simulink model "vr_octavia_graphs"  (Simulink 7.5)
settings: Solver=ode45  StartTime=0.0  StopTime=111.56  RelTol=1e-3
PostLoadFcn:
  | load octavia_testlap
undefined symbols (not defined in the file or in its folder): octavia_graphs
libraries: vrlib x26, simulink x1
Description:
  | Vehicle Dynamics Visualization with Graphs
  | 
  | This example extends the vr_octavia example and shows how combine virtual
  | reality canvas in one figure with other graphical user interface objects.
  | In this case, three graphs are displayed under the virtual scene and updated
  | in each major simulation time step.
  | 
  | The 'VR Visualization with Graphs' subsystem contains the 'octavia_graphs'
  | S-Function that provides this functionality.
settings Model: Creator=Sehnal  LastModifiedBy=Danek  ExtModeArmWhenConnect=off  BufferReuse=off
settings DataIOCC: SignalLoggingName=sigsOut
settings OptimizationCC: BooleanDataType=off  InlineInvariantSignals=on  OptimizeBlockIOStorage=off  BufferReuse=off  ExpressionFolding=off  LocalBlockOutputs=off  InitFltsAndDblsToZero=on
settings DebuggingCC: CheckExecutionContextPreStartOutputMsg=on  CheckExecutionContextRuntimeOutputMsg=on  SignalResolutionControl=TryResolveAllWithWarning  SolverPrmCheckMsg=none  MultiTaskDSMMsg=warning  MultiTaskCondExecSysMsg=none  StrictBusMsg=None
settings RTWCC: RetainRTWFile=on  ProcessScript=grt_make_rtw_hook  IncludeERTFirstTime=on
settings GRTTargetCC: TargetFcnLib=ansi_tfl_tmw.mat

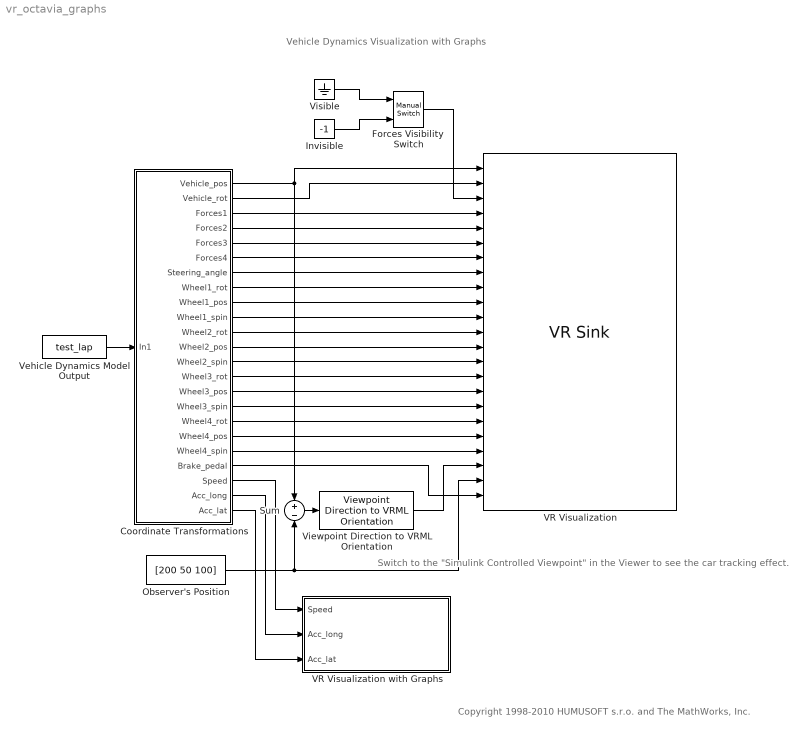
== system vr_octavia_graphs ==
  note: Vehicle Dynamics Visualization with Graphs
  note: Switch to the "Simulink Controlled Viewpoint"
      | in the Viewer to see the car tracking effect.
  note: Copyright 1998-2010 HUMUSOFT s.r.o. and The MathWorks, Inc.
  Coordinate Transformations : Subsystem
  Forces Visibility  Switch : simulink/Signal Routing/Manual Switch  SystemSampleTime=-1  sw=1  action=0  varsize=off
  Invisible : Constant  Value=-1  OutDataType=sfix(16)  OutScaling=2^0
  Observer's Position : Constant  Value=[200 50 100]  OutDataType=sfix(16)  OutScaling=2^0
  Sum : Sum  Inputs=+-  OutDataType=sfix(16)  OutScaling=2^0
  VR Visualization : vrlib/VR Sink  InstantiateOnLoad=on  SampleTime=0.04  ViewEnable=on  RemoteChange=off  RemoteView=on  FieldsWritten=Vehicle_pos_Car1.translation.3.1.double#Vehicle_rot_Car1.rotation.4.1.double#Forces_visible_Car1.whichChoice.1.1.double#Force1_Car1.scale.3.1.double#Force2_Car1.scale.3.1.double#Force3_Car1.scale.3.1.double#Force4_Car1.scale.3.1.double#SteeringWheelAngle1_Car1.rotation.4.1.double#WheelFL_Car1.rotation.4.1.double#WheelFL_Car1.translation.3.1.double#WheelSpinFL_Car1.rotation.4.1.double#WheelFR_Car1.rotation.4.1.double#WheelFR_Car1.translation.3.1.double#WheelSpinFR_Car1.rotation.4.1.double#WheelRL_Car1.rotation.4.1.double#WheelRL_Car1.translation.3.1.double#WheelSpinRL_Car1.rotation.4.1.double#WheelRR_Car1.rotation.4.1.double#WheelRR_Car1.translation.3.1.double#WheelSpinRR_Car1.rotation.4.1.double#FlyingCamera.orientation.4.1.double#FlyingCamera.position.3.1.double#Brake_Switch_Car1.whichChoice.1.1.double  WorldFileName=octavia_scene.wrl  WorldDescription=Vehicle Dynamics Visualization - Skoda Octavia  AutoView=on  VideoDimensions=[]
  VR Visualization with Graphs : Subsystem  LoadFcn=octavia_graphs([], [], [], 'LoadBlock', [], [])  StartFcn=octavia_graphs([], [], [], 'Start', [], 'octavia_scene.wrl')  StopFcn=octavia_graphs([], [], [], 'Stop', [], [])  mask(Virtual Reality Canvas with Graphs){y1range=[0 40], y2range=[-20 20], y3range=[-20 20], worldfile=octavia_scene.wrl}
      mask prompts: y1range "Speed range:"; y2range "Longitudal acceleration range:"; y3range "Latitudal acceleration range:"; worldfile "Associated VRML file:"
      mask help:
      | Block inputs - speed and longitudal and lateral accelerations are drawn
      | in three different plots in one figure together with virtual reality canvas
      | that shows the virtual world specified by the 'Associated VRML file' parameter.
      settings: CopyFcn=octavia_graphs([], [], [], 'CopyBlock', [], [])  DeleteFcn=octavia_graphs([], [], [], 'DeleteBlock', [], [])  NameChangeFcn=octavia_graphs([], [], [], 'NameChange', [], [])
      mask Display:
      | port_label('input',1,'Speed');
      | port_label('input',2,'Longitudal acceleration');
      | port_label('input',3,'Lateral acceleration')
  Vehicle Dynamics Model Output : FromWorkspace  VariableName=test_lap  SampleTime=0.04  OutputAfterFinalValue=Holding final value
  Viewpoint Direction to VRML Orientation : vrlib/Utilities/Viewpoint Direction to VRML Orientation  SystemSampleTime=-1
  Visible : Ground
  wires:
  Visible/1 -> Forces Visibility  Switch/1
  Invisible/1 -> Forces Visibility  Switch/2
  Vehicle Dynamics Model Output/1 -> Coordinate Transformations/1(In1)
  Coordinate Transformations/1(Vehicle_pos) -> VR Visualization/1, Sum/1
  Coordinate Transformations/2(Vehicle_rot) -> VR Visualization/2
  Forces Visibility  Switch/1 -> VR Visualization/3
  Coordinate Transformations/3(Forces1) -> VR Visualization/4
  Coordinate Transformations/4(Forces2) -> VR Visualization/5
  Coordinate Transformations/5(Forces3) -> VR Visualization/6
  Coordinate Transformations/6(Forces4) -> VR Visualization/7
  Coordinate Transformations/7(Steering_angle) -> VR Visualization/8
  Coordinate Transformations/8(Wheel1_rot) -> VR Visualization/9
  Coordinate Transformations/9(Wheel1_pos) -> VR Visualization/10
  Coordinate Transformations/10(Wheel1_spin) -> VR Visualization/11
  Coordinate Transformations/11(Wheel2_rot) -> VR Visualization/12
  Coordinate Transformations/12(Wheel2_pos) -> VR Visualization/13
  Coordinate Transformations/13(Wheel2_spin) -> VR Visualization/14
  Coordinate Transformations/14(Wheel3_rot) -> VR Visualization/15
  Coordinate Transformations/15(Wheel3_pos) -> VR Visualization/16
  Coordinate Transformations/16(Wheel3_spin) -> VR Visualization/17
  Coordinate Transformations/17(Wheel4_rot) -> VR Visualization/18
  Coordinate Transformations/18(Wheel4_pos) -> VR Visualization/19
  Coordinate Transformations/19(Wheel4_spin) -> VR Visualization/20
  Coordinate Transformations/20(Brake_pedal) -> VR Visualization/23
  Sum/1 -> Viewpoint Direction to VRML Orientation/1
  Viewpoint Direction to VRML Orientation/1 -> VR Visualization/21
  Observer's Position/1 -> VR Visualization/22, Sum/2
  Coordinate Transformations/21(Speed) -> VR Visualization with Graphs/1(Speed)
  Coordinate Transformations/23(Acc_lat) -> VR Visualization with Graphs/3(Acc_lat)
  Coordinate Transformations/22(Acc_long) -> VR Visualization with Graphs/2(Acc_long)

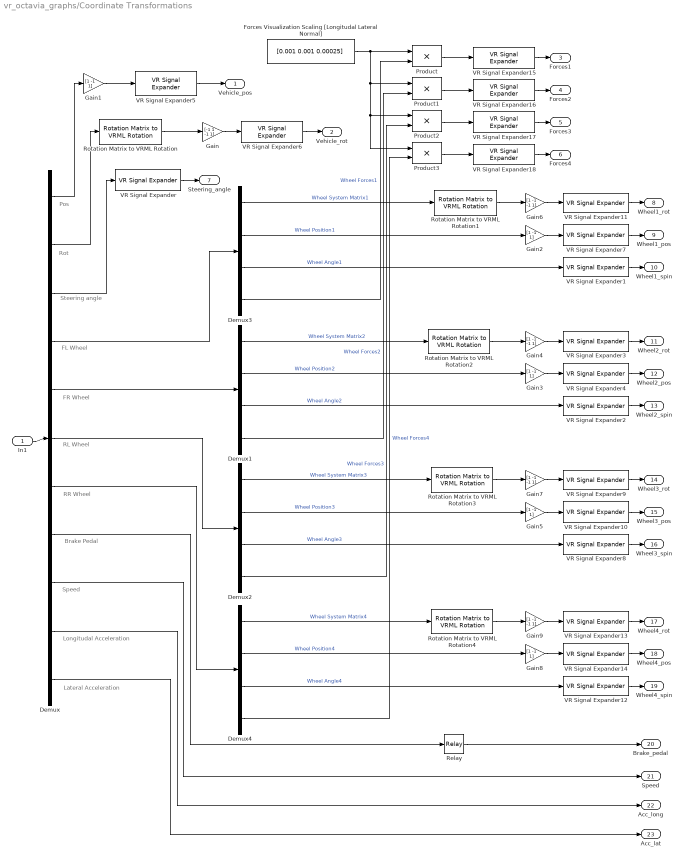
== system vr_octavia_graphs/Coordinate Transformations ==
  note: Steering angle
  note: FL Wheel
  note: FR Wheel
  note: RL Wheel
  note: RR Wheel
  note: Brake Pedal
  note: Pos
  note: Rot
  note: Speed
  note: Longitudal Acceleration
  note: Lateral Acceleration
  In1 : Inport  OutDataType=sfix(16)  OutScaling=2^0
  Demux : Demux  Outputs=[3,9,1,16,16,16,16,1,1,1,1]
  Demux{1..4} (4 alike) : Demux  Outputs=[9,3,1,3]
  Forces Visualization Scaling [Longitudal Lateral Normal] : Constant  Value=[0.001 0.001 0.00025]  OutDataType=sfix(16)  OutScaling=2^0
  Gain : Gain  Gain=[-1 1 -1 1]  ParameterDataType=sfix(16)  ParameterScaling=2^0  OutDataType=sfix(16)  OutScaling=2^0  SaturateOnIntegerOverflow=on  OutDataTypeStr=Inherit: Same as input  ParamDataTypeStr=Inherit: Same as input
  Gain{1..3,5,8} (5 alike) : Gain  Gain=[1 -1 1]  ParameterDataType=sfix(16)  ParameterScaling=2^0  OutDataType=sfix(16)  OutScaling=2^0  SaturateOnIntegerOverflow=on  OutDataTypeStr=Inherit: Same as input  ParamDataTypeStr=Inherit: Same as input
  Gain{4,6..7,9} (4 alike) : Gain  Gain=[1 -1 -1 1]  ParameterDataType=sfix(16)  ParameterScaling=2^0  OutDataType=sfix(16)  OutScaling=2^0  SaturateOnIntegerOverflow=on  OutDataTypeStr=Inherit: Same as input  ParamDataTypeStr=Inherit: Same as input
  Product{,1..3} (4 alike) : Product  OutDataType=sfix(16)  OutScaling=2^0  SaturateOnIntegerOverflow=on  OutDataTypeStr=Inherit: Same as first input
  Relay : Relay  OutDataType=sfix(16)  OutScaling=2^0
  Rotation Matrix to VRML Rotation{,1..4} (5 alike) : vrlib/Utilities/Rotation Matrix to VRML Rotation  SystemSampleTime=-1  maxzero=1e-12
  VR Signal Expander{,1..2,8,12} (5 alike) : vrlib/VR Signal Expander  SystemSampleTime=-1  outwidth=4  outidx=[4]
  VR Signal Expander{4,7,10,14} (4 alike) : vrlib/VR Signal Expander  SystemSampleTime=-1  outwidth=3  outidx=[1 3 2 ]
  VR Signal Expander{3,6,9,11,13} (5 alike) : vrlib/VR Signal Expander  SystemSampleTime=-1  outwidth=4  outidx=[1 3 2 4]
  VR Signal Expander{5,15..18} (5 alike) : vrlib/VR Signal Expander  SystemSampleTime=-1  outwidth=3  outidx=[1 3 2]
  Vehicle_pos : Outport  OutDataType=sfix(16)  OutScaling=2^0
  Vehicle_rot : Outport  Port=2  OutDataType=sfix(16)  OutScaling=2^0
  Forces1 : Outport  Port=3  OutDataType=sfix(16)  OutScaling=2^0
  Forces2 : Outport  Port=4  OutDataType=sfix(16)  OutScaling=2^0
  Forces3 : Outport  Port=5  OutDataType=sfix(16)  OutScaling=2^0
  Forces4 : Outport  Port=6  OutDataType=sfix(16)  OutScaling=2^0
  Steering_angle : Outport  Port=7  OutDataType=sfix(16)  OutScaling=2^0
  Wheel1_rot : Outport  Port=8  OutDataType=sfix(16)  OutScaling=2^0
  Wheel1_pos : Outport  Port=9  OutDataType=sfix(16)  OutScaling=2^0
  Wheel1_spin : Outport  Port=10  OutDataType=sfix(16)  OutScaling=2^0
  Wheel2_rot : Outport  Port=11  OutDataType=sfix(16)  OutScaling=2^0
  Wheel2_pos : Outport  Port=12  OutDataType=sfix(16)  OutScaling=2^0
  Wheel2_spin : Outport  Port=13  OutDataType=sfix(16)  OutScaling=2^0
  Wheel3_rot : Outport  Port=14  OutDataType=sfix(16)  OutScaling=2^0
  Wheel3_pos : Outport  Port=15  OutDataType=sfix(16)  OutScaling=2^0
  Wheel3_spin : Outport  Port=16  OutDataType=sfix(16)  OutScaling=2^0
  Wheel4_rot : Outport  Port=17  OutDataType=sfix(16)  OutScaling=2^0
  Wheel4_pos : Outport  Port=18  OutDataType=sfix(16)  OutScaling=2^0
  Wheel4_spin : Outport  Port=19  OutDataType=sfix(16)  OutScaling=2^0
  Brake_pedal : Outport  Port=20  OutDataType=sfix(16)  OutScaling=2^0
  Speed : Outport  Port=21  OutDataType=sfix(16)  OutScaling=2^0
  Acc_long : Outport  Port=22  OutDataType=sfix(16)  OutScaling=2^0
  Acc_lat : Outport  Port=23  OutDataType=sfix(16)  OutScaling=2^0
  wires:
  Gain1/1 -> VR Signal Expander5/1
  Rotation Matrix to VRML Rotation/1 -> Gain/1
  Gain/1 -> VR Signal Expander6/1
  Gain6/1 -> VR Signal Expander11/1
  Gain2/1 -> VR Signal Expander7/1
  Demux3/1 -> Rotation Matrix to VRML Rotation1/1  "Wheel System Matrix1"
  Demux3/2 -> Gain2/1  "Wheel Position1"
  Demux3/3 -> VR Signal Expander1/1  "Wheel Angle1"
  Gain4/1 -> VR Signal Expander3/1
  Rotation Matrix to VRML Rotation2/1 -> Gain4/1
  Gain3/1 -> VR Signal Expander4/1
  Demux1/1 -> Rotation Matrix to VRML Rotation2/1  "Wheel System Matrix2"
  Demux1/2 -> Gain3/1  "Wheel Position2"
  Demux1/3 -> VR Signal Expander2/1  "Wheel Angle2"
  Gain7/1 -> VR Signal Expander9/1
  Rotation Matrix to VRML Rotation3/1 -> Gain7/1
  Demux2/4 -> Product2/2  "Wheel Forces3"
  Gain5/1 -> VR Signal Expander10/1
  Demux2/1 -> Rotation Matrix to VRML Rotation3/1  "Wheel System Matrix3"
  Demux2/2 -> Gain5/1  "Wheel Position3"
  Demux2/3 -> VR Signal Expander8/1  "Wheel Angle3"
  Gain9/1 -> VR Signal Expander13/1
  Rotation Matrix to VRML Rotation4/1 -> Gain9/1
  Demux4/4 -> Product3/2  "Wheel Forces4"
  Gain8/1 -> VR Signal Expander14/1
  Demux4/1 -> Rotation Matrix to VRML Rotation4/1  "Wheel System Matrix4"
  Demux4/2 -> Gain8/1  "Wheel Position4"
  Demux4/3 -> VR Signal Expander12/1  "Wheel Angle4"
  VR Signal Expander5/1 -> Vehicle_pos/1
  Demux3/4 -> Product/2  "Wheel Forces1"
  Demux1/4 -> Product1/2  "Wheel Forces2"
  Product/1 -> VR Signal Expander15/1
  Product1/1 -> VR Signal Expander16/1
  Product2/1 -> VR Signal Expander17/1
  Product3/1 -> VR Signal Expander18/1
  VR Signal Expander6/1 -> Vehicle_rot/1
  VR Signal Expander15/1 -> Forces1/1
  VR Signal Expander16/1 -> Forces2/1
  VR Signal Expander17/1 -> Forces3/1
  VR Signal Expander18/1 -> Forces4/1
  VR Signal Expander/1 -> Steering_angle/1
  VR Signal Expander11/1 -> Wheel1_rot/1
  In1/1 -> Demux/1
  VR Signal Expander7/1 -> Wheel1_pos/1
  VR Signal Expander1/1 -> Wheel1_spin/1
  VR Signal Expander3/1 -> Wheel2_rot/1
  VR Signal Expander4/1 -> Wheel2_pos/1
  VR Signal Expander2/1 -> Wheel2_spin/1
  VR Signal Expander9/1 -> Wheel3_rot/1
  VR Signal Expander10/1 -> Wheel3_pos/1
  VR Signal Expander8/1 -> Wheel3_spin/1
  VR Signal Expander13/1 -> Wheel4_rot/1
  VR Signal Expander14/1 -> Wheel4_pos/1
  VR Signal Expander12/1 -> Wheel4_spin/1
  Demux/8 -> Relay/1
  Relay/1 -> Brake_pedal/1
  Demux/1 -> Gain1/1
  Demux/2 -> Rotation Matrix to VRML Rotation/1
  Demux/3 -> VR Signal Expander/1
  Demux/4 -> Demux3/1
  Demux/5 -> Demux1/1
  Demux/6 -> Demux2/1
  Demux/7 -> Demux4/1
  Forces Visualization Scaling [Longitudal Lateral Normal]/1 -> Product/1, Product1/1, Product2/1, Product3/1
  Rotation Matrix to VRML Rotation1/1 -> Gain6/1
  Demux/9 -> Speed/1
  Demux/10 -> Acc_long/1
  Demux/11 -> Acc_lat/1

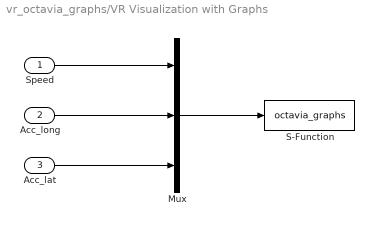
== system vr_octavia_graphs/VR Visualization with Graphs ==
  Speed : Inport  OutDataType=fixdt(1, 16)  OutScaling=2^0
  Acc_long : Inport  Port=2  OutDataType=fixdt(1, 16)  OutScaling=2^0
  Acc_lat : Inport  Port=3  OutDataType=fixdt(1, 16)  OutScaling=2^0
  Mux : Mux  Inputs=3
  S-Function : S-Function  FunctionName=octavia_graphs  Parameters=[y1range y2range y3range], worldfile  EnableBusSupport=off
  wires:
  Speed/1 -> Mux/1
  Acc_long/1 -> Mux/2
  Acc_lat/1 -> Mux/3
  Mux/1 -> S-Function/1
